simulink model "controller_poleplace"  (R2015a)
settings: Solver=ode3  StartTime=0  StopTime=inf  FixedStep=sampleTime_qcsim  MaxStep=0.1  RelTol=1e-3
InitFcn:
  | % load parameters of the default quadrotor
  | disp('Quadrotor parameters loaded by InitFcn')
  | paramsControl %load mdl_quadcopter as well!
undefined symbols (not defined in the file or in its folder): controlParams, quad, quadEDT
libraries: simulink x1
settings Model: CovSFcnEnable=off  Creator=corkep  LastModifiedBy=ra
settings DataIOCC: LimitDataPoints=off  SaveFormat=StructureWithTime  SignalLoggingSaveFormat=ModelDataLogs  SignalLogging=off  DSMLogging=off
settings OptimizationCC: ExpressionDepthLimit=2147483647  OptimizeModelRefInitCode=on  LifeSpan=1
settings DebuggingCC: UnderspecifiedInitializationDetection=Classic  MergeDetectMultiDrivingBlocksExec=none  SolverPrmCheckMsg=warning  FcnCallInpInsideContextMsg=UseLocalSettings  StateNameClashWarn=warning
settings HardwareCC: TargetBitPerLong=64  TargetBitPerPointer=64  TargetLongLongMode=on  TargetIntDivRoundTo=Zero  TargetEndianess=LittleEndian  TargetWordSize=64  TargetHWDeviceType=MATLAB Host  ProdEqTarget=off
settings RTWCC: SystemTargetFile=ert_shrlib.tlc  GenCodeOnly=on  MakeCommand="make_rtw OPTS=\"-DDEFAULT_BUFFER_SIZE=4600\""  GenerateMakefile=off  TemplateMakefile=ert_default_tmf  Description=Embedded Coder (host-based shared library target)  BuildConfiguration=Faster Runs  RTWCompilerOptimization=on
settings CodeAppCC: IgnoreCustomStorageClasses=off
settings STFCustomTargetCC: ParMdlRefBuildCompliant=on  CompOptLevelCompliant=on  IncludeMdlTerminateFcn=off  CombineOutputUpdateFcns=on  MatFileLogging=on  MultiInstanceERTCode=on  CodeInterfacePackaging=Reusable function  SupportContinuousTime=off  SupportVariableSizeSignals=off  ModelStepFunctionPrototypeControlCompliant=on  SystemTargetFile=ert_shrlib.tlc
settings ERTTargetCC: ParMdlRefBuildCompliant=on  CompOptLevelCompliant=on  IncludeMdlTerminateFcn=off  MatFileLogging=on  MultiInstanceERTCode=on  CodeInterfacePackaging=Reusable function  SupportContinuousTime=off  SupportVariableSizeSignals=off  ModelStepFunctionPrototypeControlCompliant=on  MultiInstanceErrorCode=Warning  ERTCustomFileTemplate=example_file_process.tlc

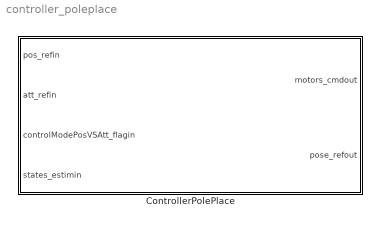
== system controller_poleplace ==
  ControllerPolePlace : Subsystem  TreatAsAtomicUnit=on

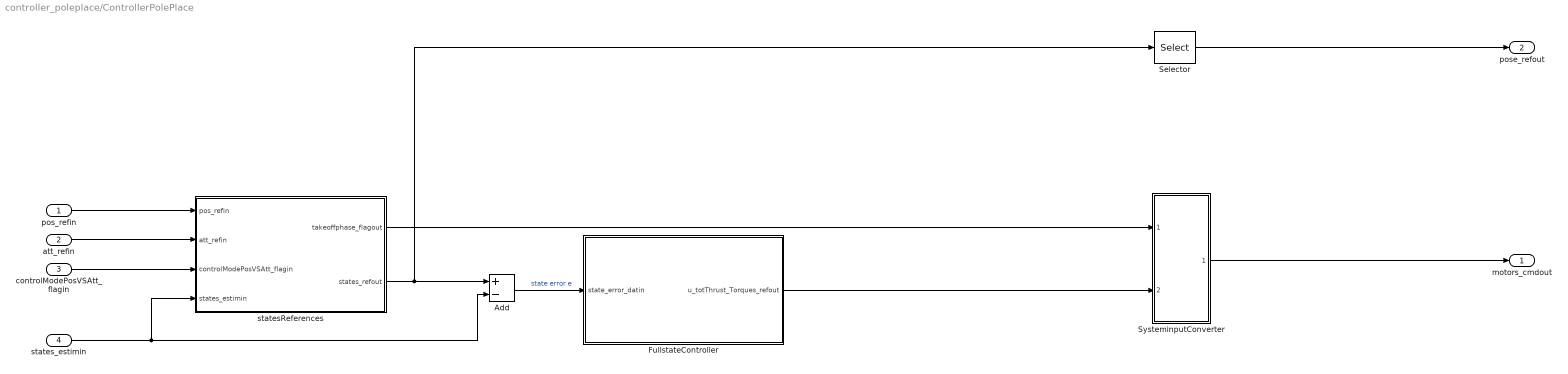
== system controller_poleplace/ControllerPolePlace ==
  pos_refin : Inport
  att_refin : Inport  Port=2
  controlModePosVSAtt_flagin : Inport  Port=3
  states_estimin : Inport  Port=4
  Add : Sum  Inputs=+-
  FullstateController : Subsystem
  Selector : Selector  InputPortWidth=12  Indices=[1:6]
  SysteminputConverter : Subsystem
  statesReferences : Subsystem
  motors_cmdout : Outport
  pose_refout : Outport  Port=2
  wires:
  Selector/1 -> pose_refout/1
  statesReferences/2(states_refout) -> Add/1, Selector/1
  controlModePosVSAtt_flagin/1 -> statesReferences/3(controlModePosVSAtt_flagin)
  states_estimin/1 -> statesReferences/4(states_estimin), Add/2
  att_refin/1 -> statesReferences/2(att_refin)
  pos_refin/1 -> statesReferences/1(pos_refin)
  Add/1 -> FullstateController/1(state_error_datin)  "state error e"
  statesReferences/1(takeoffphase_flagout) -> SysteminputConverter/1(takeoffphase_flagin)
  FullstateController/1(u_totThrust_Torques_refout) -> SysteminputConverter/2(u_totThrust_Torques_refin)
  SysteminputConverter/1(motors_cmdout) -> motors_cmdout/1

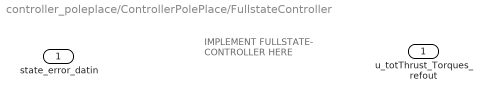
== system controller_poleplace/ControllerPolePlace/FullstateController ==
  note: IMPLEMENT FULLSTATE-
      | CONTROLLER HERE
  state_error_datin : Inport
  u_totThrust_Torques_refout : Outport

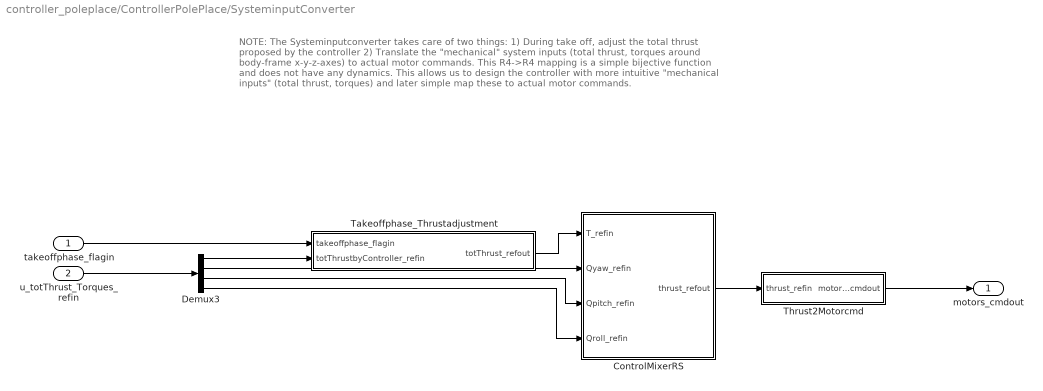
== system controller_poleplace/ControllerPolePlace/SysteminputConverter ==
  note: NOTE: The Systeminputconverter takes care of two things:
      | 1) During take off, adjust the total thrust proposed by the controller
      | 2) Translate the "mechanical" system inputs (total thrust, torques around body-frame x-y-z-axes) to actual motor commands.
      | This R4->R4 mapping is a simple bijective function and does not have any dynamics. This allows us to design the controller with more intuitive "mechanical inputs" (total thrust, torques) and later simple map these to actual motor commands.
  takeoffphase_flagin : Inport
  u_totThrust_Torques_refin : Inport  Port=2
  ControlMixerRS : Subsystem
  Demux3 : Demux
  Takeoffphase_Thrustadjustment : Subsystem
  Thrust2Motorcmd : Subsystem
  motors_cmdout : Outport
  wires:
  takeoffphase_flagin/1 -> Takeoffphase_Thrustadjustment/1(takeoffphase_flagin)
  Takeoffphase_Thrustadjustment/1(totThrust_refout) -> ControlMixerRS/1(T_refin)
  Demux3/1 -> Takeoffphase_Thrustadjustment/2(totThrustbyController_refin)
  u_totThrust_Torques_refin/1 -> Demux3/1
  Demux3/4 -> ControlMixerRS/4(Qroll_refin)
  Demux3/3 -> ControlMixerRS/3(Qpitch_refin)
  Demux3/2 -> ControlMixerRS/2(Qyaw_refin)
  ControlMixerRS/1(thrust_refout) -> Thrust2Motorcmd/1(thrust_refin)
  Thrust2Motorcmd/1(motors_cmdout) -> motors_cmdout/1

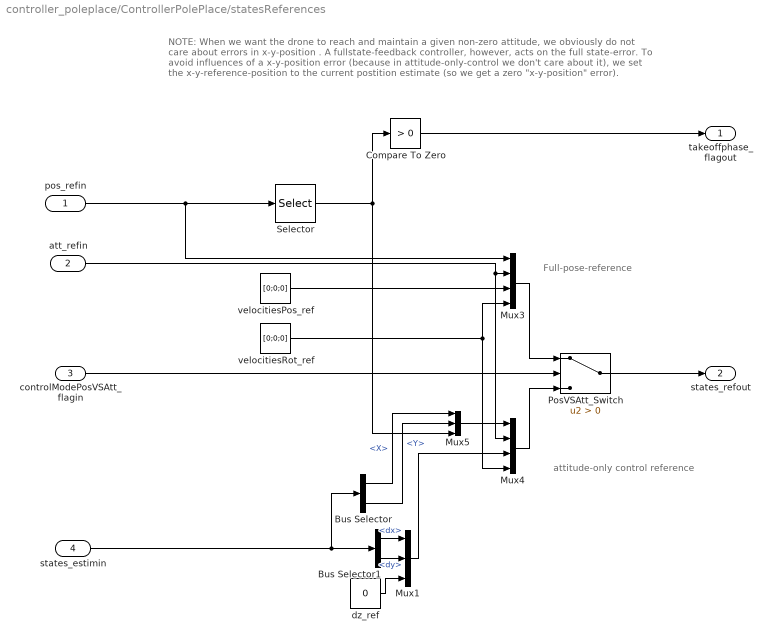
== system controller_poleplace/ControllerPolePlace/statesReferences ==
  note: attitude-only control reference
  note: Full-pose-reference
  note: NOTE: When we want the drone to reach and maintain a given non-zero attitude,
      | we obviously do not care about errors in x-y-position . A fullstate-feedback controller, however, acts
      | on the full state-error. To avoid influences of a x-y-position error (because in attitude-only-control we don't care about it),
      | we set the x-y-reference-position to the current postition estimate (so we get a zero "x-y-position" error).
  pos_refin : Inport
  att_refin : Inport  Port=2
  controlModePosVSAtt_flagin : Inport  Port=3
  states_estimin : Inport  Port=4
  Bus Selector : BusSelector  OutputSignals=X,Y
  Bus Selector1 : BusSelector  OutputSignals=dx,dy
  Compare To Zero : simulink/Logic and Bit Operations/Compare To Zero  relop=>  OutDataTypeStr=boolean
  Mux1 : Mux  Inputs=3
  Mux3 : Mux
  Mux4 : Mux
  Mux5 : Mux  Inputs=3
  PosVSAtt_Switch : Switch  Criteria=u2 > Threshold
  Selector : Selector  InputPortWidth=3  Indices=[3]
  dz_ref : Constant  Value=0
  velocitiesPos_ref : Constant  Value=[0;0;0]
  velocitiesRot_ref : Constant  Value=[0;0;0]
  takeoffphase_flagout : Outport
  states_refout : Outport  Port=2
  wires:
  dz_ref/1 -> Mux1/3
  Mux1/1 -> Mux4/3
  Bus Selector1/2 -> Mux1/2  "<dy>"
  Bus Selector1/1 -> Mux1/1  "<dx>"
  Mux5/1 -> Mux4/1
  Mux4/1 -> PosVSAtt_Switch/3
  Bus Selector/2 -> Mux5/2  "<Y>"
  Bus Selector/1 -> Mux5/1  "<X>"
  Mux3/1 -> PosVSAtt_Switch/1
  controlModePosVSAtt_flagin/1 -> PosVSAtt_Switch/2
  Selector/1 -> Compare To Zero/1, Mux5/3
  PosVSAtt_Switch/1 -> states_refout/1
  velocitiesRot_ref/1 -> Mux4/4, Mux3/4
  velocitiesPos_ref/1 -> Mux3/3
  states_estimin/1 -> Bus Selector/1, Bus Selector1/1
  att_refin/1 -> Mux4/2, Mux3/2
  pos_refin/1 -> Mux3/1, Selector/1
  Compare To Zero/1 -> takeoffphase_flagout/1

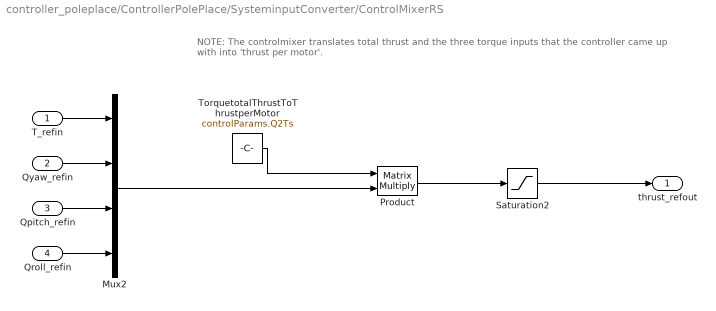
== system controller_poleplace/ControllerPolePlace/SysteminputConverter/ControlMixerRS ==
  note: NOTE: The controlmixer translates total thrust and the three torque inputs that the controller came up with into 'thrust per motor'.
  T_refin : Inport
  Qyaw_refin : Inport  Port=2
  Qpitch_refin : Inport  Port=3
  Qroll_refin : Inport  Port=4
  Mux2 : Mux
  Product : Product  Multiplication=Matrix(*)  RndMeth=Zero
  Saturation2 : Saturate  UpperLimit=-0.0118  LowerLimit=-0.3235
  TorquetotalThrustToThrustperMotor : Constant  Value=controlParams.Q2Ts
  thrust_refout : Outport
  wires:
  Qroll_refin/1 -> Mux2/4
  Qpitch_refin/1 -> Mux2/3
  Qyaw_refin/1 -> Mux2/2
  T_refin/1 -> Mux2/1
  Product/1 -> Saturation2/1
  TorquetotalThrustToThrustperMotor/1 -> Product/1
  Mux2/1 -> Product/2
  Saturation2/1 -> thrust_refout/1

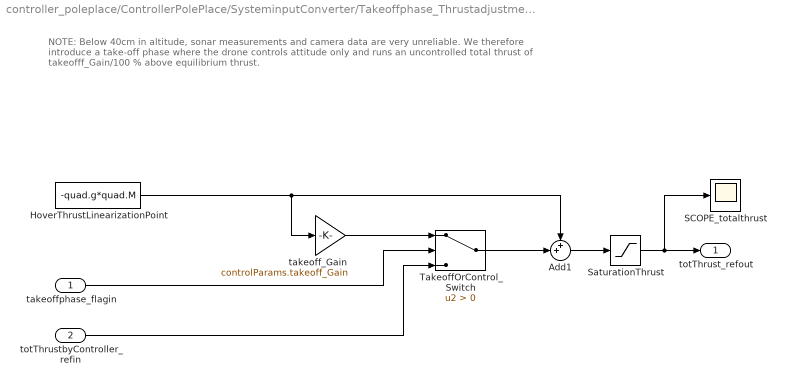
== system controller_poleplace/ControllerPolePlace/SysteminputConverter/Takeoffphase_Thrustadjustment ==
  note: NOTE: Below 40cm in altitude, sonar measurements and camera data are very unreliable.
      | We therefore introduce a take-off phase where the drone controls attitude only and runs an uncontrolled total thrust of takeofff_Gain/100  % above equilibrium thrust.
  takeoffphase_flagin : Inport
  totThrustbyController_refin : Inport  Port=2
  Add1 : Sum  Inputs=++|
  HoverThrustLinearizationPoint : Constant  Value=-quad.g*quad.M
  "SCOPE_totalthrust " : Scope
  SaturationThrust : Saturate  UpperLimit=controlParams.totalThrust_maxRelative*controlParams.motorsThrust_i_UpperLimit*4  LowerLimit=-(controlParams.totalThrust_maxRelative*controlParams.motorsThrust_i_UpperLimit*4)
  TakeoffOrControl_Switch : Switch  Criteria=u2 > Threshold
  takeoff_Gain : Gain  Gain=controlParams.takeoff_Gain
  totThrust_refout : Outport
  wires:
  takeoffphase_flagin/1 -> TakeoffOrControl_Switch/2
  SaturationThrust/1 -> totThrust_refout/1, "SCOPE_totalthrust "/1
  TakeoffOrControl_Switch/1 -> Add1/2
  takeoff_Gain/1 -> TakeoffOrControl_Switch/1
  HoverThrustLinearizationPoint/1 -> Add1/1, takeoff_Gain/1
  totThrustbyController_refin/1 -> TakeoffOrControl_Switch/3
  Add1/1 -> SaturationThrust/1

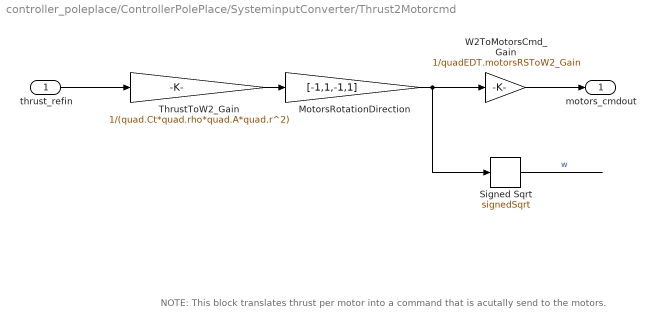
== system controller_poleplace/ControllerPolePlace/SysteminputConverter/Thrust2Motorcmd ==
  note: NOTE: This block translates thrust per motor into a command that is acutally send to the motors.
  thrust_refin : Inport
  MotorsRotationDirection : Gain  Gain=[-1,1,-1,1]
  Signed Sqrt : Sqrt  Operator=signedSqrt  SaturateOnIntegerOverflow=on
  ThrustToW2_Gain : Gain  Gain=1/(quad.Ct*quad.rho*quad.A*quad.r^2)
  W2ToMotorsCmd_Gain : Gain  Gain=1/quadEDT.motorsRSToW2_Gain
  motors_cmdout : Outport
  wires:
  MotorsRotationDirection/1 -> W2ToMotorsCmd_Gain/1, Signed Sqrt/1
  Signed Sqrt/1 -> ?  "w"
  W2ToMotorsCmd_Gain/1 -> motors_cmdout/1
  thrust_refin/1 -> ThrustToW2_Gain/1
  ThrustToW2_Gain/1 -> MotorsRotationDirection/1
